simulink model "f14_airframe"  (R2015a)
settings: Solver=ode45  StartTime=0.0  StopTime=10.0  MaxStep=0.1  RelTol=1e-3
undefined symbols (not defined in the file): Md, Mq, Mw, Uo, Zd
settings Model: ModifiedByFormat=The MathWorks Inc.  CovSFcnEnable=off  Creator=The MathWorks Inc.  LastModifiedBy=The MathWorks Inc.
settings ConfigSet: ConfigType=Model
settings SolverCC: Priority=auto
settings DataIOCC: SaveOutput=off  SaveTime=off  SignalLoggingName=f14_airframe
settings OptimizationCC: InlineParams=on  InlineParamsCompatibleMode=off  ExpressionDepthLimit=2147483647  InitFltsAndDblsToZero=on  ForceBlockIOInitOptimize=off  EvaledLifeSpan=1  SimCompilerOptimization=Off
settings DebuggingCC: SaveWithParameterizedLinksMsg=none  UnderspecifiedInitializationDetection=Classic  MergeDetectMultiDrivingBlocksExec=none  SignalResolutionControl=TryResolveAllWithWarning  SolverPrmCheckMsg=warning  MultiTaskDSMMsg=warning  MultiTaskCondExecSysMsg=none  FcnCallInpInsideContextMsg=UseLocalSettings  AllowSymbolicDim=off  StateNameClashWarn=warning  SFMismatchInSimAndRtwBecauseOfMissingDataTypeDiag=warning
settings RTWCC: EnableTagging=off  RTWCompilerOptimization=Off
settings CodeAppCC: ParameterTuningSideEffectCode=Output function  AllmanStyle=off
settings GRTTargetCC: TargetFcnLib=ansi_tfl_tmw.mat  CombineOutputUpdateFcns=off  EnableShiftOperators=off  PortableWordSizesTransition=off  GenerateErtSFunctionTransition=off  CreateSILPILBlockTransition=None  CodeProfilingSaveOptionsTransition=SummaryOnly  CodeExecutionProfilingTransition=off  CodeProfilingInstrumentationTransition=off  CodeExecutionProfileVariableTransition=executionProfile  GRTInterface=on

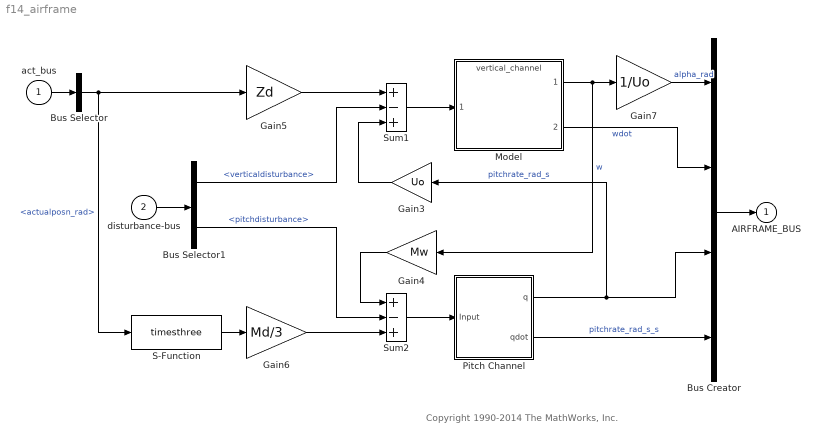
== system f14_airframe ==
  note: Copyright 1990-2014 The MathWorks, Inc.
  act_bus : Inport  IOType=none  Commented=off  StatePerturbationForJacobian=1.0e-05  OutDataTypeStr=Bus: ACT_BUS
  disturbance-bus : Inport  IOType=none  Commented=off  StatePerturbationForJacobian=1.0e-05  Port=2  OutDataTypeStr=Bus: DISTURB_BUS
  Bus Creator : BusCreator  IOType=none  Commented=off  StatePerturbationForJacobian=1.0e-05  Inputs='alpha_rad','wdot','pitchrate_rad_s','pitchrate_rad_s_s'  OutDataTypeStr=Bus: AIRFRAME_BUS
  Bus Selector : BusSelector  IOType=none  Commented=off  StatePerturbationForJacobian=1.0e-05  OutputSignals=actualposn_rad
  Bus Selector1 : BusSelector  IOType=none  Commented=off  StatePerturbationForJacobian=1.0e-05  OutputSignals=verticaldisturbance,pitchdisturbance
  Gain3 : Gain  IOType=none  Commented=off  StatePerturbationForJacobian=1.0e-05  Gain=Uo  SaturateOnIntegerOverflow=on  OutDataTypeStr=Inherit: Same as input  ParamDataTypeStr=Inherit: Same as input
  Gain4 : Gain  IOType=none  Commented=off  StatePerturbationForJacobian=1.0e-05  Gain=Mw  SaturateOnIntegerOverflow=on  OutDataTypeStr=Inherit: Same as input  ParamDataTypeStr=Inherit: Same as input
  Gain5 : Gain  IOType=none  Commented=off  StatePerturbationForJacobian=1.0e-05  Gain=Zd  SaturateOnIntegerOverflow=on  OutDataTypeStr=Inherit: Same as input  ParamDataTypeStr=Inherit: Same as input
  Gain6 : Gain  IOType=none  Commented=off  StatePerturbationForJacobian=1.0e-05  Gain=Md/3  SaturateOnIntegerOverflow=on  OutDataTypeStr=Inherit: Same as input  ParamDataTypeStr=Inherit: Same as input
  Gain7 : Gain  IOType=none  Commented=off  StatePerturbationForJacobian=1.0e-05  Gain=1/Uo  SaturateOnIntegerOverflow=on  OutDataTypeStr=Inherit: Same as input  ParamDataTypeStr=Inherit: Same as input
  Model : ModelReference  IOType=none  Commented=off  StatePerturbationForJacobian=1.0e-05  ModelNameDialog=vertical_channel  SimulationMode=Normal  ModelReferenceVersion=1.12  CopyOfModelName=vertical_channel  DefaultDataLogging=on
  Pitch Channel : Subsystem  IOType=none  Commented=off  StatePerturbationForJacobian=1.0e-05
  S-Function : S-Function  IOType=none  Commented=off  StatePerturbationForJacobian=1.0e-05  FunctionName=timesthree
  Sum1 : Sum  IOType=none  Commented=off  StatePerturbationForJacobian=1.0e-05  Inputs=+-+  SaturateOnIntegerOverflow=on  InputSameDT=on  OutDataTypeStr=Inherit: Same as first input
  Sum2 : Sum  IOType=none  Commented=off  StatePerturbationForJacobian=1.0e-05  Inputs=+-+  SaturateOnIntegerOverflow=on  InputSameDT=on  OutDataTypeStr=Inherit: Same as first input
  AIRFRAME_BUS : Outport  IOType=none  Commented=off  StatePerturbationForJacobian=1.0e-05  OutDataTypeStr=Bus: AIRFRAME_BUS  InitialOutput=0  BusOutputAsStruct=on
  wires:
  Gain4/1 -> Sum2/1
  Gain3/1 -> Sum1/3
  Gain7/1 -> Bus Creator/1  "alpha_rad"
  Bus Selector1/1 -> Sum1/2  "<verticaldisturbance>"
  Sum2/1 -> Pitch Channel/1(Input)
  Bus Selector1/2 -> Sum2/2  "<pitchdisturbance>"
  Gain5/1 -> Sum1/1
  Gain6/1 -> Sum2/3
  Sum1/1 -> Model/1
  Model/1 -> Gain7/1, Gain4/1  "w"
  Model/2 -> Bus Creator/2  "wdot"
  Pitch Channel/1(q) -> Gain3/1, Bus Creator/3  "pitchrate_rad_s"
  Pitch Channel/2(qdot) -> Bus Creator/4  "pitchrate_rad_s_s"
  act_bus/1 -> Bus Selector/1
  Bus Selector/1 -> Gain5/1, S-Function/1  "<actualposn_rad>"
  Bus Creator/1 -> AIRFRAME_BUS/1
  disturbance-bus/1 -> Bus Selector1/1
  S-Function/1 -> Gain6/1

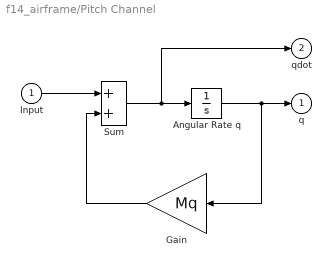
== system f14_airframe/Pitch Channel ==
  Input : Inport  IOType=none  Commented=off  StatePerturbationForJacobian=1.0e-05
  "Angular Rate q " : Integrator  IOType=none  Commented=off  StatePerturbationForJacobian=1.0e-05
  Gain : Gain  IOType=none  Commented=off  StatePerturbationForJacobian=1.0e-05  Gain=Mq  SaturateOnIntegerOverflow=on  OutDataTypeStr=Inherit: Same as input  ParamDataTypeStr=Inherit: Same as input
  Sum : Sum  IOType=none  Commented=off  StatePerturbationForJacobian=1.0e-05  SaturateOnIntegerOverflow=on  InputSameDT=on  OutDataTypeStr=Inherit: Same as first input
  q : Outport  IOType=none  Commented=off  StatePerturbationForJacobian=1.0e-05
  qdot : Outport  IOType=none  Commented=off  StatePerturbationForJacobian=1.0e-05  Port=2
  wires:
  Sum/1 -> qdot/1, "Angular Rate q "/1
  "Angular Rate q "/1 -> Gain/1, q/1
  Gain/1 -> Sum/2
  Input/1 -> Sum/1
